simulink model "IEEE9BusSystem_1_1"  (R2025a)
settings: Solver=FixedStepDiscrete  StartTime=0.0  StopTime=20  FixedStep=Ts  RelTol=1e-3  AbsTol=1e-3  EnableMultiTasking=on
PreLoadFcn:
  | Ts = 1/60;
libraries: ee_lib x50, nesl_utility x29, fl_lib x22, eeGeneralControl x6, eeSmAC1C x3, eeSmPSS1A x3
(part 1 of 2)
Description:
  | IEEE 9-Bus System
settings Model: Creator=The MathWorks, Inc.  LastModifiedBy=Vishal
settings SolverCC: AutoScaleAbsTol=off  AlgebraicLoopSolver=TrustRegion
settings DataIOCC: MaxDataPoints=110000  SaveOutput=off  DSMLogging=off  SaveTime=off  ReturnWorkspaceOutputs=off  SignalLoggingName=logsout_IEEE9BusLoadflow
settings OptimizationCC: ReuseModelBlockBuffer=off  LifeSpan=inf
settings DebuggingCC: UnderspecifiedInitializationDetection=Classic  MergeDetectMultiDrivingBlocksExec=none  MaxConsecutiveZCsMsg=warning  UnconnectedInputMsg=warning  UnconnectedOutputMsg=warning  UnconnectedLineMsg=warning  SFUnexpectedBacktrackingDiag=warning  SFNoUnconditionalDefaultTransitionDiag=warning  SFExecutionAtInitializationDiag=none  ArithmeticOperatorsInVariantConditions=warning
settings ModelReferenceCC: EnableRefExpFcnMdlSchedulingChecks=on
settings SFSimCC: SimUseLocalCustomCode=off
settings RTWCC: RTWUseLocalCustomCode=off  GPUComputeCapability=3.5
settings CodeAppCC: StateflowObjectComments=on
settings GRTTargetCC: TargetLangStandard=C89/C90 (ANSI)
settings ConfigComp: CovMetricSettings=dw  CovSaveCumulativeToWorkspaceVar=on  CovSaveSingleToWorkspaceVar=on  CovExternalEMLEnable=off
settings SimscapeCC: SimscapeNormalizeSystem=off  SimscapeLogType=all  SimscapeLogName=simlog_IEEE9BusSystem  SimscapeLogLimitData=off  SimscapeOperatingPoint=op

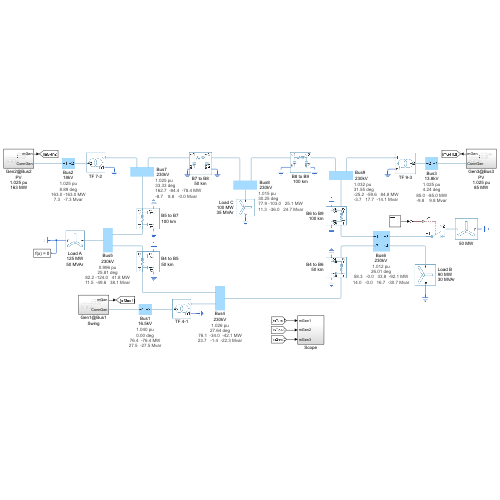
[thumbnail: Simulink's stored preview of the top-level diagram]
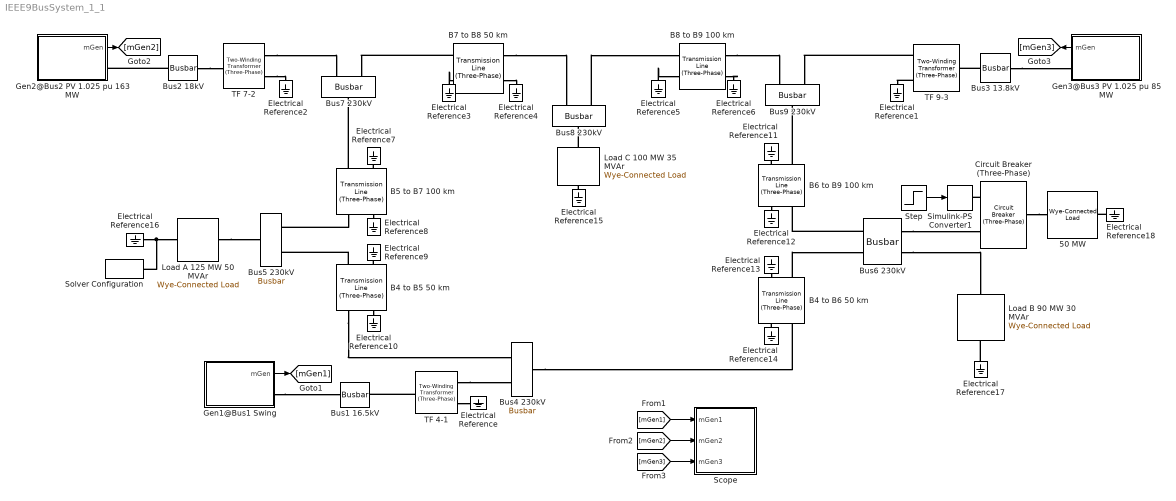
== system IEEE9BusSystem_1_1 ==
  50 MW : ee_lib/Passive/RLC Assemblies/Wye-Connected Load  port_option=ee.enum.threePhasePort.composite  parameterization=2  component_structure=1  component_structure_PQ=1  R=1 Ohm  L=0.001 H  C=1e-6 F  VRated=230 kV  FRated=60 Hz  P=50 MW  Qpos=30e6 V*A  Qneg=-100 V*A  R_parasitic=1e-6 Ohm  G_parasitic=1e-6 1/Ohm  R_parasitic_PQ=1e-6 Ohm  G_parasitic_PQ=1e-6*0 1/Ohm  Vmag0=230e3 V  Vang0=0 rad  Freq0=60 Hz  IL_specify=on  IL_priority=High  IL=[ 0 0 0 ] A  IL_nominal_specify=off  IL_nominal_value=1  IL_nominal_unit=A  VC_specify=on  VC_priority=High  VC=[ 0 0 0 ] V  VC_nominal_specify=off  VC_nominal_value=1  VC_nominal_unit=V
  B4 to B5 50 km : ee_lib/Passive/Lines/Transmission Line (Three-Phase)  length=50 km  freq=60 Hz  R=0.199333 Ohm/km  L=2.9658 mH/km  M=0.5803 mH/km  Cl=3.300e-3 uF/km  Cg=7.751e-3 uF/km  Rm=0.093533 Ohm/km  ModelTwoSections=ee.enum.enable.no  N=1  InterfacePosition=1 km  N1sec=1  N2sec=1  Access_ground=ee.enum.enable.no  R_parasitic=1e-6 Ohm  G_parasitic=1e-6 1/Ohm
      settings: InternalSimscapePortConfiguration="{\"Bottom\":[],\"Left\":[{\"id\":\"N1\",\"label\":\"~1\",\"type\":\"foundation.electrical.three_phase\"},{\"id\":\"g1\",\"label\":\"g1\",\"type\":\"foundation.electrical.electrical\"}],\"Right\":[{\"id\":\"N2\",\"label\":\"~2\",\"type\":\"foundation.electrical.three_phase\"},{\"id\":\"g2\",\"label\":\"g2\",\"type\":\"foundation.electrical.electrical\"}],\"Top\":[]}"
  B4 to B6 50 km : ee_lib/Passive/Lines/Transmission Line (Three-Phase)  length=50 km  freq=60 Hz  R=0.248707 Ohm/km  L=3.0967 mH/km  M=0.5148 mH/km  Cl=2.698e-3 uF/km  Cg=7.751e-3 uF/km  Rm=0.068847 Ohm/km  ModelTwoSections=ee.enum.enable.no  N=1  InterfacePosition=1 km  N1sec=1  N2sec=1  Access_ground=ee.enum.enable.no  R_parasitic=1e-6 Ohm  G_parasitic=1e-6 1/Ohm
      settings: InternalSimscapePortConfiguration="{\"Bottom\":[],\"Left\":[{\"id\":\"N1\",\"label\":\"~1\",\"type\":\"foundation.electrical.three_phase\"},{\"id\":\"g1\",\"label\":\"g1\",\"type\":\"foundation.electrical.electrical\"}],\"Right\":[{\"id\":\"N2\",\"label\":\"~2\",\"type\":\"foundation.electrical.three_phase\"},{\"id\":\"g2\",\"label\":\"g2\",\"type\":\"foundation.electrical.electrical\"}],\"Top\":[]}"
  B5 to B7 100 km : ee_lib/Passive/Lines/Transmission Line (Three-Phase)  length=100 km  freq=60 Hz  R=0.24165 Ohm/km  L=2.8816 mH/km  M=0.6224 mH/km  Cl=2.531e-3 uF/km  Cg=7.751e-3 uF/km  Rm=0.07237 Ohm/km  ModelTwoSections=ee.enum.enable.no  N=1  InterfacePosition=1 km  N1sec=1  N2sec=1  Access_ground=ee.enum.enable.no  R_parasitic=1e-6 Ohm  G_parasitic=1e-6 1/Ohm
      settings: InternalSimscapePortConfiguration="{\"Bottom\":[],\"Left\":[{\"id\":\"N1\",\"label\":\"~1\",\"type\":\"foundation.electrical.three_phase\"},{\"id\":\"g1\",\"label\":\"g1\",\"type\":\"foundation.electrical.electrical\"}],\"Right\":[{\"id\":\"N2\",\"label\":\"~2\",\"type\":\"foundation.electrical.three_phase\"},{\"id\":\"g2\",\"label\":\"g2\",\"type\":\"foundation.electrical.electrical\"}],\"Top\":[]}"
  B6 to B9 100 km : ee_lib/Passive/Lines/Transmission Line (Three-Phase)  length=100 km  freq=60 Hz  R=0.26634 Ohm/km  L=2.9658 mH/km  M=0.5803 mH/km  Cl=3.400e-3 uF/km  Cg=7.751e-3 uF/km  Rm=0.06003 Ohm/km  ModelTwoSections=ee.enum.enable.no  N=1  InterfacePosition=1 km  N1sec=1  N2sec=1  Access_ground=ee.enum.enable.no  R_parasitic=1e-6 Ohm  G_parasitic=1e-6 1/Ohm
      settings: InternalSimscapePortConfiguration="{\"Bottom\":[],\"Left\":[{\"id\":\"N1\",\"label\":\"~1\",\"type\":\"foundation.electrical.three_phase\"},{\"id\":\"g1\",\"label\":\"g1\",\"type\":\"foundation.electrical.electrical\"}],\"Right\":[{\"id\":\"N2\",\"label\":\"~2\",\"type\":\"foundation.electrical.three_phase\"},{\"id\":\"g2\",\"label\":\"g2\",\"type\":\"foundation.electrical.electrical\"}],\"Top\":[]}"
  B7 to B8 50 km : ee_lib/Passive/Lines/Transmission Line (Three-Phase)  length=50 km  freq=60 Hz  R=0.18875 Ohm/km  L=2.7226 mH/km  M=0.7019 mH/km  Cl=2.731e-3 uF/km  Cg=6.751e-3 uF/km  Rm=0.09882 Ohm/km  ModelTwoSections=ee.enum.enable.no  N=1  InterfacePosition=1 km  N1sec=1  N2sec=1  Access_ground=ee.enum.enable.no  R_parasitic=1e-6 Ohm  G_parasitic=1e-6 1/Ohm
      settings: InternalSimscapePortConfiguration="{\"Bottom\":[],\"Left\":[{\"id\":\"N1\",\"label\":\"~1\",\"type\":\"foundation.electrical.three_phase\"},{\"id\":\"g1\",\"label\":\"g1\",\"type\":\"foundation.electrical.electrical\"}],\"Right\":[{\"id\":\"N2\",\"label\":\"~2\",\"type\":\"foundation.electrical.three_phase\"},{\"id\":\"g2\",\"label\":\"g2\",\"type\":\"foundation.electrical.electrical\"}],\"Top\":[]}"
  B8 to B9 100 km : ee_lib/Passive/Lines/Transmission Line (Three-Phase)  length=100 km  freq=60 Hz  R=0.17077 Ohm/km  L=2.3184 mH/km  M=0.9040 mH/km  Cl=9.097e-4 uF/km  Cg=7.751e-3 uF/km  Rm=0.10782 Ohm/km  ModelTwoSections=ee.enum.enable.no  N=1  InterfacePosition=1 km  N1sec=1  N2sec=1  Access_ground=ee.enum.enable.no  R_parasitic=1e-6 Ohm  G_parasitic=1e-6 1/Ohm
      settings: InternalSimscapePortConfiguration="{\"Bottom\":[],\"Left\":[{\"id\":\"N1\",\"label\":\"~1\",\"type\":\"foundation.electrical.three_phase\"},{\"id\":\"g1\",\"label\":\"g1\",\"type\":\"foundation.electrical.electrical\"}],\"Right\":[{\"id\":\"N2\",\"label\":\"~2\",\"type\":\"foundation.electrical.three_phase\"},{\"id\":\"g2\",\"label\":\"g2\",\"type\":\"foundation.electrical.electrical\"}],\"Top\":[]}"
  Bus1 16.5kV : ee_lib/Connectors & References/Busbar  Tag="1.040 pu\\n0.00 deg\\n76.4  -76.4 MW\\n27.5  -27.5 Mvar"  n_nodes=ee.enum.connectors.busbar_number_of_connections.two  VRated=16.5 kV  freq=60 Hz  show_ps=ee.enum.connectors.busbar_measurement.false
      settings: AttributesFormatString=%<Tag>  InternalSimscapePortConfiguration="{\"Bottom\":[],\"Left\":[{\"id\":\"N1\",\"label\":\"~1\",\"type\":\"foundation.electrical.three_phase\"}],\"Right\":[{\"id\":\"N2\",\"label\":\"~2\",\"type\":\"foundation.electrical.three_phase\"}],\"Top\":[]}"
  Bus2 18kV : ee_lib/Connectors & References/Busbar  Tag="1.025 pu\\n8.89 deg\\n163.0 -163.0 MW\\n7.3   -7.3 Mvar"  n_nodes=ee.enum.connectors.busbar_number_of_connections.two  VRated=18 kV  freq=60 Hz  show_ps=ee.enum.connectors.busbar_measurement.false
      settings: AttributesFormatString=%<Tag>  InternalSimscapePortConfiguration="{\"Bottom\":[],\"Left\":[{\"id\":\"N1\",\"label\":\"~1\",\"type\":\"foundation.electrical.three_phase\"}],\"Right\":[{\"id\":\"N2\",\"label\":\"~2\",\"type\":\"foundation.electrical.three_phase\"}],\"Top\":[]}"
  Bus3 13.8kV : ee_lib/Connectors & References/Busbar  Tag="1.025 pu\\n4.24 deg\\n85.0  -85.0 MW\\n-9.8    9.8 Mvar"  n_nodes=ee.enum.connectors.busbar_number_of_connections.two  VRated=13.8 kV  freq=60 Hz  show_ps=ee.enum.connectors.busbar_measurement.false
      settings: AttributesFormatString=%<Tag>  InternalSimscapePortConfiguration="{\"Bottom\":[],\"Left\":[{\"id\":\"N1\",\"label\":\"~1\",\"type\":\"foundation.electrical.three_phase\"}],\"Right\":[{\"id\":\"N2\",\"label\":\"~2\",\"type\":\"foundation.electrical.three_phase\"}],\"Top\":[]}"
  Bus4 230kV : ee_lib/Connectors & References/Busbar  Tag="1.026 pu\\n27.64 deg\\n76.1  -34.0  -42.1 MW\\n23.7   -1.4  -22.3 Mvar"  n_nodes=ee.enum.connectors.busbar_number_of_connections.three  VRated=230 kV  freq=60 Hz  show_ps=ee.enum.connectors.busbar_measurement.false
      settings: AttributesFormatString=%<Tag>  InternalSimscapePortConfiguration="{\"Bottom\":[],\"Left\":[{\"id\":\"N1\",\"label\":\"~1\",\"type\":\"foundation.electrical.three_phase\"},{\"id\":\"N3\",\"label\":\"~3\",\"type\":\"foundation.electrical.three_phase\"}],\"Right\":[{\"id\":\"N2\",\"label\":\"~2\",\"type\":\"foundation.electrical.three_phase\"}],\"Top\":[]}"
  Bus5 230kV : ee_lib/Connectors & References/Busbar  Tag="0.996 pu\\n25.81 deg\\n82.2 -124.0   41.8 MW\\n11.5  -49.6   38.1 Mvar"  n_nodes=ee.enum.connectors.busbar_number_of_connections.three  VRated=230 kV  freq=60 Hz  show_ps=ee.enum.connectors.busbar_measurement.false
      settings: AttributesFormatString=%<Tag>  InternalSimscapePortConfiguration="{\"Bottom\":[],\"Left\":[{\"id\":\"N1\",\"label\":\"~1\",\"type\":\"foundation.electrical.three_phase\"},{\"id\":\"N3\",\"label\":\"~3\",\"type\":\"foundation.electrical.three_phase\"}],\"Right\":[{\"id\":\"N2\",\"label\":\"~2\",\"type\":\"foundation.electrical.three_phase\"}],\"Top\":[]}"
  Bus6 230kV : ee_lib/Connectors & References/Busbar  Tag="1.012 pu\\n26.01 deg\\n58.3   -0.0   33.8  -92.1 MW\\n14.0   -0.0   16.7  -30.7 Mvar"  n_nodes=ee.enum.connectors.busbar_number_of_connections.four  VRated=230 kV  freq=60 Hz  show_ps=ee.enum.connectors.busbar_measurement.false
      settings: AttributesFormatString=%<Tag>  InternalSimscapePortConfiguration="{\"Bottom\":[],\"Left\":[{\"id\":\"N1\",\"label\":\"~1\",\"type\":\"foundation.electrical.three_phase\"},{\"id\":\"N3\",\"label\":\"~3\",\"type\":\"foundation.electrical.three_phase\"}],\"Right\":[{\"id\":\"N2\",\"label\":\"~2\",\"type\":\"foundation.electrical.three_phase\"},{\"id\":\"N4\",\"label\":\"~4\",\"type\":\"foundation.electrical.three_phase\"}],\"Top\":[]}"
  Bus7 230kV : ee_lib/Connectors & References/Busbar  Tag="1.025 pu\\n33.33 deg\\n162.7  -84.4  -78.4 MW\\n-8.7    8.8   -0.0 Mvar"  n_nodes=ee.enum.connectors.busbar_number_of_connections.three  VRated=230 kV  freq=60 Hz  show_ps=ee.enum.connectors.busbar_measurement.false
      settings: AttributesFormatString=%<Tag>  InternalSimscapePortConfiguration="{\"Bottom\":[],\"Left\":[{\"id\":\"N1\",\"label\":\"~1\",\"type\":\"foundation.electrical.three_phase\"},{\"id\":\"N3\",\"label\":\"~3\",\"type\":\"foundation.electrical.three_phase\"}],\"Right\":[{\"id\":\"N2\",\"label\":\"~2\",\"type\":\"foundation.electrical.three_phase\"}],\"Top\":[]}"
  Bus8 230kV : ee_lib/Connectors & References/Busbar  Tag="1.015 pu\\n30.25 deg\\n77.9 -103.0   25.1 MW\\n11.3  -36.0   24.7 Mvar"  n_nodes=ee.enum.connectors.busbar_number_of_connections.three  VRated=230 kV  freq=60 Hz  show_ps=ee.enum.connectors.busbar_measurement.false
      settings: AttributesFormatString=%<Tag>  InternalSimscapePortConfiguration="{\"Bottom\":[],\"Left\":[{\"id\":\"N1\",\"label\":\"~1\",\"type\":\"foundation.electrical.three_phase\"},{\"id\":\"N3\",\"label\":\"~3\",\"type\":\"foundation.electrical.three_phase\"}],\"Right\":[{\"id\":\"N2\",\"label\":\"~2\",\"type\":\"foundation.electrical.three_phase\"}],\"Top\":[]}"
  Bus9 230kV : ee_lib/Connectors & References/Busbar  Tag="1.032 pu\\n31.55 deg\\n-25.2  -59.6   84.8 MW\\n-3.7   17.7  -14.1 Mvar"  n_nodes=ee.enum.connectors.busbar_number_of_connections.three  VRated=230 kV  freq=60 Hz  show_ps=ee.enum.connectors.busbar_measurement.false
      settings: AttributesFormatString=%<Tag>  InternalSimscapePortConfiguration="{\"Bottom\":[],\"Left\":[{\"id\":\"N1\",\"label\":\"~1\",\"type\":\"foundation.electrical.three_phase\"},{\"id\":\"N3\",\"label\":\"~3\",\"type\":\"foundation.electrical.three_phase\"}],\"Right\":[{\"id\":\"N2\",\"label\":\"~2\",\"type\":\"foundation.electrical.three_phase\"}],\"Top\":[]}"
  Circuit Breaker (Three-Phase) : ee_lib/Switches & Breakers/Circuit Breaker (Three-Phase)  R_closed=0.001 Ohm  G_open=1e-8 1/Ohm  threshold=0.5 V  breaker_behavior=ee.enum.switches.breakerBehavior.zeroCrossingDisable
      settings: InternalSimscapePortConfiguration="{\"Bottom\":[],\"Left\":[{\"id\":\"vT\",\"label\":\"vT\",\"type\":\"input\"},{\"id\":\"N1\",\"label\":\"~1\",\"type\":\"foundation.electrical.three_phase\"}],\"Right\":[{\"id\":\"N2\",\"label\":\"~2\",\"type\":\"foundation.electrical.three_phase\"}],\"Top\":[]}"
  Electrical Reference{,1..18} (19 alike) : fl_lib/Electrical/Electrical Elements/Electrical Reference
  Gen1@Bus1 Swing : Subsystem
  Gen2@Bus2 PV 1.025 pu 163 MW : Subsystem
  Gen3@Bus3 PV 1.025 pu 85 MW : Subsystem
  Load A 125 MW 50 MVAr : ee_lib/Passive/RLC Assemblies/Wye-Connected Load  port_option=ee.enum.threePhasePort.composite  parameterization=2  component_structure=1  component_structure_PQ=4  R=1 Ohm  L=0.001 H  C=1e-6 F  VRated=230e3 V  FRated=60 Hz  P=125e6 W  Qpos=50e6 V*A  Qneg=-100 V*A  R_parasitic=1e-6 Ohm  G_parasitic=1e-6 1/Ohm  R_parasitic_PQ=1e-6 Ohm  G_parasitic_PQ=1e-6 1/Ohm  Vmag0=230e3 V  Vang0=0 deg  Freq0=60 Hz  IL_specify=on  IL_priority=High  IL=[ 0 0 0 ] A  IL_nominal_specify=off  IL_nominal_value=1  IL_nominal_unit=A  VC_specify=on  VC_priority=High  VC=[ 0 0 0 ] V  VC_nominal_specify=off  VC_nominal_value=1  VC_nominal_unit=V
  Load B 90 MW 30 MVAr : ee_lib/Passive/RLC Assemblies/Wye-Connected Load  port_option=ee.enum.threePhasePort.composite  parameterization=2  component_structure=1  component_structure_PQ=4  R=1 Ohm  L=0.001 H  C=1e-6 F  VRated=230e3 V  FRated=60 Hz  P=90e6 W  Qpos=30e6 V*A  Qneg=-100 V*A  R_parasitic=1e-6 Ohm  G_parasitic=1e-6 1/Ohm  R_parasitic_PQ=1e-6 Ohm  G_parasitic_PQ=1e-6*0 1/Ohm  Vmag0=230e3 V  Vang0=0 deg  Freq0=60 Hz  IL_specify=on  IL_priority=High  IL=[ 0 0 0 ] A  IL_nominal_specify=off  IL_nominal_value=1  IL_nominal_unit=A  VC_specify=on  VC_priority=High  VC=[ 0 0 0 ] V  VC_nominal_specify=off  VC_nominal_value=1  VC_nominal_unit=V
  Load C 100 MW 35 MVAr : ee_lib/Passive/RLC Assemblies/Wye-Connected Load  port_option=ee.enum.threePhasePort.composite  parameterization=2  component_structure=1  component_structure_PQ=4  R=1 Ohm  L=0.001 H  C=1e-6 F  VRated=230e3 V  FRated=60 Hz  P=100e6 W  Qpos=35e6 V*A  Qneg=-100 V*A  R_parasitic=1e-6 Ohm  G_parasitic=1e-6 1/Ohm  R_parasitic_PQ=1e-6 Ohm  G_parasitic_PQ=1e-6 1/Ohm  Vmag0=230e3 V  Vang0=0 deg  Freq0=60 Hz  IL_specify=on  IL_priority=High  IL=[ 0 0 0 ] A  IL_nominal_specify=off  IL_nominal_value=1  IL_nominal_unit=A  VC_specify=on  VC_priority=High  VC=[ 0 0 0 ] V  VC_nominal_specify=off  VC_nominal_value=1  VC_nominal_unit=V
  Scope : Subsystem
  Simulink-PS Converter1 : nesl_utility/Simulink-PS Converter  PhysicalDomain=network_engine_domain  SubClassName=ps_input  LeftPortType=input  RightPortType=output  PseudoPeriodic=off  Frequencies=[]  NoiseDistribution=none  NoiseParameters=[]  Unit=1  AffineConversion=off  FilteringAndDerivatives=provide  SimscapeFilterOrder=1  InputFilterTimeConstant=0.001  UdotUserProvided=0
  Solver Configuration : nesl_utility/Solver Configuration  PhysicalDomain=network_engine_domain  SubClassName=solver  LeftPortType=input  RightPortType=generic  Tones=[]  Harmonics=[]  SimulateNoise=off  Profile=off  UseLocalSampling=off  EnableSwitchedLinearOptims=on  FrequencyDomain=off  UseCCode=off  RelTol=0.001  AbsTol=1e-06  MinStep=1e-09  ToWorkspace=off  RevertToSquareIcSolve=off  NumHomotopyIterations=100  PhasorMode=off  PhasorModeNumHarmonics=1  ConsistencySolver=NEWTON_FTOL  IndexReductionMethod=DerivativeReplacement  DoDC=off  ResidualTolerance=1e-09  ConsistencyTolSource=GLOBAL  ConsistencyAbsTol=0.001  ConsistencyRelTol=0.001  ConsistencyTolFactor=0.001  UseLocalSolver=on  LocalSolverChoice=NE_BACKWARD_EULER_ADVANCER  ResolveIndetEquations=on  FunctionEvalNumThread=1  LocalSolverSampleTime=Ts  DoFixedCost=on  MaxNonlinIter=3  MaxModeIter=2  ComputeImpulses=off  ImpulseIterations=2  LinearAlgebra=auto  LinearAlgebraNumThread=0  EquationFormulation=NE_FREQUENCY_TIME_EF  DelaysMemoryBudget=1024  AutomaticFiltering=on  FilteringTimeConstant=0.001  PartitionStorageMethod=AS_NEEDED  PartitionMemoryBudget=1024  PartitionMethod=FAST  MultibodyUseLocalSolver=off  MultibodyLocalSolverChoice=ODE1  MultibodyLocalSolverSampleTime=0.001
  Step : Step  Time=10  Before=1  After=0  SampleTime=0
  TF 4-1 : ee_lib/Passive/Transformers/Two-Winding Transformer (Three-Phase)  SRated=100e6 V*A  FRated=60 Hz  Winding1Connection=ee.enum.windingconnection.Yn  VRated1=230e3 V  Winding2Connection=ee.enum.windingconnection.delta1  VRated2=16.5e3 V  CoreType=ee.enum.coretype.fivelimb  pu_Rw1=1e-4  pu_Rw2=1e-4  leakage_reactance_option=ee.enum.transformer_leakage.include  pu_Xl1=0.0576/2  pu_Xl2=0.0576/2  magnetizing_resistance_option=ee.enum.transformer_magnetizingResistance.include  pu_Rm=500  magnetizing_reactance_option=ee.enum.transformer_magnetizingReactance.include  saturation_option=ee.enum.transformer_saturation.exclude  pu_Xm=500  current_data=[0, .002, 1, 2]  magnetic_flux_data=[0, 1.2, 1.5, 1.51]  pu_X0=0.5  i1_specify=off  i1_priority=None  i1=[ 0 0 0 ] A  i1_nominal_specify=off  i1_nominal_value=1  i1_nominal_unit=A  i2_specify=off  i2_priority=None  i2=[ 0 0 0 ] A  i2_nominal_specify=off  i2_nominal_value=1  i2_nominal_unit=A  phi_specify=off  phi_priority=None  phi=[ 0 0 0 ]  phi_nominal_specify=off  phi_nominal_value=1  phi_nominal_unit=1  power_dissipated_specify=off  power_dissipated_priority=None  power_dissipated=0 W  power_dissipated_nominal_specify=off  power_dissipated_nominal_value=1  power_dissipated_nominal_unit=W
      settings: InternalSimscapePortConfiguration="{\"Bottom\":[],\"Left\":[{\"id\":\"N1\",\"label\":\"~1\",\"type\":\"foundation.electrical.three_phase\"},{\"id\":\"n1\",\"label\":\"n1\",\"type\":\"foundation.electrical.electrical\"}],\"Right\":[{\"id\":\"N2\",\"label\":\"~2\",\"type\":\"foundation.electrical.three_phase\"}],\"Top\":[]}"
  TF 7-2 : ee_lib/Passive/Transformers/Two-Winding Transformer (Three-Phase)  SRated=100e6 V*A  FRated=60 Hz  Winding1Connection=ee.enum.windingconnection.Yn  VRated1=230e3 V  Winding2Connection=ee.enum.windingconnection.delta1  VRated2=18e3 V  CoreType=ee.enum.coretype.fivelimb  pu_Rw1=1e-4  pu_Rw2=1e-4  leakage_reactance_option=ee.enum.transformer_leakage.include  pu_Xl1=0.0625/2  pu_Xl2=0.0625/2  magnetizing_resistance_option=ee.enum.transformer_magnetizingResistance.include  pu_Rm=500  magnetizing_reactance_option=ee.enum.transformer_magnetizingReactance.include  saturation_option=ee.enum.transformer_saturation.exclude  pu_Xm=500  current_data=[0, .002, 1, 2]  magnetic_flux_data=[0, 1.2, 1.5, 1.51]  pu_X0=0.5  i1_specify=off  i1_priority=None  i1=[ 0 0 0 ] A  i1_nominal_specify=off  i1_nominal_value=1  i1_nominal_unit=A  i2_specify=off  i2_priority=None  i2=[ 0 0 0 ] A  i2_nominal_specify=off  i2_nominal_value=1  i2_nominal_unit=A  phi_specify=off  phi_priority=None  phi=[ 0 0 0 ]  phi_nominal_specify=off  phi_nominal_value=1  phi_nominal_unit=1  power_dissipated_specify=off  power_dissipated_priority=None  power_dissipated=0 W  power_dissipated_nominal_specify=off  power_dissipated_nominal_value=1  power_dissipated_nominal_unit=W
      settings: InternalSimscapePortConfiguration="{\"Bottom\":[],\"Left\":[{\"id\":\"N1\",\"label\":\"~1\",\"type\":\"foundation.electrical.three_phase\"},{\"id\":\"n1\",\"label\":\"n1\",\"type\":\"foundation.electrical.electrical\"}],\"Right\":[{\"id\":\"N2\",\"label\":\"~2\",\"type\":\"foundation.electrical.three_phase\"}],\"Top\":[]}"
  TF 9-3 : ee_lib/Passive/Transformers/Two-Winding Transformer (Three-Phase)  SRated=100e6 V*A  FRated=60 Hz  Winding1Connection=ee.enum.windingconnection.Yn  VRated1=230e3 V  Winding2Connection=ee.enum.windingconnection.delta1  VRated2=13.8e3 V  CoreType=ee.enum.coretype.fivelimb  pu_Rw1=1e-4  pu_Rw2=1e-4  leakage_reactance_option=ee.enum.transformer_leakage.include  pu_Xl1=0.0586/2  pu_Xl2=0.0586/2  magnetizing_resistance_option=ee.enum.transformer_magnetizingResistance.include  pu_Rm=500  magnetizing_reactance_option=ee.enum.transformer_magnetizingReactance.include  saturation_option=ee.enum.transformer_saturation.exclude  pu_Xm=500  current_data=[0, .002, 1, 2]  magnetic_flux_data=[0, 1.2, 1.5, 1.51]  pu_X0=0.5  i1_specify=off  i1_priority=None  i1=[ 0 0 0 ] A  i1_nominal_specify=off  i1_nominal_value=1  i1_nominal_unit=A  i2_specify=off  i2_priority=None  i2=[ 0 0 0 ] A  i2_nominal_specify=off  i2_nominal_value=1  i2_nominal_unit=A  phi_specify=off  phi_priority=None  phi=[ 0 0 0 ]  phi_nominal_specify=off  phi_nominal_value=1  phi_nominal_unit=1  power_dissipated_specify=off  power_dissipated_priority=None  power_dissipated=0 W  power_dissipated_nominal_specify=off  power_dissipated_nominal_value=1  power_dissipated_nominal_unit=W
      settings: InternalSimscapePortConfiguration="{\"Bottom\":[],\"Left\":[{\"id\":\"N1\",\"label\":\"~1\",\"type\":\"foundation.electrical.three_phase\"},{\"id\":\"n1\",\"label\":\"n1\",\"type\":\"foundation.electrical.electrical\"}],\"Right\":[{\"id\":\"N2\",\"label\":\"~2\",\"type\":\"foundation.electrical.three_phase\"}],\"Top\":[]}"
  wires:
  Gen2@Bus2 PV 1.025 pu 163 MW/1(mGen) -> [mGen2]
  Gen1@Bus1 Swing/1(mGen) -> [mGen1]
  Gen3@Bus3 PV 1.025 pu 85 MW/1(mGen) -> [mGen3]
  Step/1 -> Simulink-PS Converter1/1
  [mGen1] -> Scope/1(mGen1)
  [mGen2] -> Scope/2(mGen2)
  [mGen3] -> Scope/3(mGen3)
  connections:
  Electrical Reference16/LConn1 -- Solver Configuration/RConn1 -- Load A 125 MW 50 MVAr/RConn1
  B6 to B9 100 km/RConn1 -- Bus9 230kV/RConn1
  B8 to B9 100 km/RConn1 -- Bus9 230kV/LConn1
  B7 to B8 50 km/RConn1 -- Bus8 230kV/LConn1
  B4 to B5 50 km/RConn1 -- Bus5 230kV/LConn2
  B5 to B7 100 km/LConn1 -- Bus5 230kV/LConn1
  Load A 125 MW 50 MVAr/LConn1 -- Bus5 230kV/RConn1
  B5 to B7 100 km/RConn1 -- Bus7 230kV/RConn1
  TF 7-2/LConn1 -- Bus7 230kV/LConn1
  B6 to B9 100 km/LConn2 -- Electrical Reference12/LConn1
  TF 4-1/LConn1 -- Bus4 230kV/LConn1
  Load C 100 MW 35 MVAr/LConn1 -- Bus8 230kV/RConn1
  Electrical Reference5/LConn1 -- B8 to B9 100 km/LConn2
  B7 to B8 50 km/RConn2 -- Electrical Reference4/LConn1
  Bus8 230kV/LConn2 -- B8 to B9 100 km/LConn1
  TF 7-2/LConn2 -- Electrical Reference2/LConn1
  TF 9-3/LConn1 -- Bus9 230kV/LConn2
  TF 4-1/LConn2 -- Electrical Reference/LConn1
  B5 to B7 100 km/RConn2 -- Electrical Reference7/LConn1
  B5 to B7 100 km/LConn2 -- Electrical Reference8/LConn1
  B8 to B9 100 km/RConn2 -- Electrical Reference6/LConn1
  TF 9-3/LConn2 -- Electrical Reference1/LConn1
  B4 to B5 50 km/RConn2 -- Electrical Reference9/LConn1
  Electrical Reference3/LConn1 -- B7 to B8 50 km/LConn2
  B4 to B5 50 km/LConn2 -- Electrical Reference10/LConn1
  Electrical Reference17/LConn1 -- Load B 90 MW 30 MVAr/RConn1
  B7 to B8 50 km/LConn1 -- Bus7 230kV/LConn2
  Electrical Reference15/LConn1 -- Load C 100 MW 35 MVAr/RConn1
  Bus4 230kV/RConn1 -- B4 to B6 50 km/LConn1
  B4 to B5 50 km/LConn1 -- Bus4 230kV/LConn2
  TF 4-1/RConn1 -- Bus1 16.5kV/RConn1
  Electrical Reference14/LConn1 -- B4 to B6 50 km/LConn2
  Electrical Reference13/LConn1 -- B4 to B6 50 km/RConn2
  Bus2 18kV/RConn1 -- TF 7-2/RConn1
  Bus6 230kV/LConn1 -- B6 to B9 100 km/LConn1
  B6 to B9 100 km/RConn2 -- Electrical Reference11/LConn1
  Bus2 18kV/LConn1 -- Gen2@Bus2 PV 1.025 pu 163 MW/RConn1
  Gen1@Bus1 Swing/RConn1 -- Bus1 16.5kV/LConn1
  Bus6 230kV/RConn2 -- Load B 90 MW 30 MVAr/LConn1
  Circuit Breaker (Three-Phase)/LConn1 -- Simulink-PS Converter1/RConn1
  Electrical Reference18/LConn1 -- 50 MW/RConn1
  Circuit Breaker (Three-Phase)/RConn1 -- 50 MW/LConn1
  Bus6 230kV/RConn1 -- Circuit Breaker (Three-Phase)/LConn2
  B4 to B6 50 km/RConn1 -- Bus6 230kV/LConn2
  Bus3 13.8kV/LConn1 -- Gen3@Bus3 PV 1.025 pu 85 MW/RConn1
  Bus3 13.8kV/RConn1 -- TF 9-3/RConn1

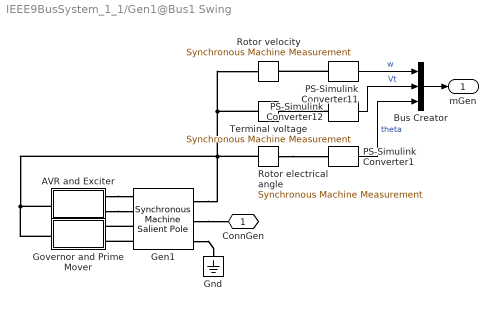
== system IEEE9BusSystem_1_1/Gen1@Bus1 Swing ==
  AVR and Exciter : Subsystem
  Bus Creator : BusCreator  Inputs=3
  Gen1 : ee_lib/Electromechanical/Synchronous/Synchronous Machine Salient Pole  port_option=ee.enum.threePhasePort.composite  SRated=247.5 MW  VRated=16.5 kV  FRated=60 Hz  nPolePairs=20  param_option=ee.enum.sm.parameterization.standard  fieldCircuitParameterization_option=ee.enum.sm.fieldparameterization.current  baseEfd=100 V  baseIfd=100 A  zero_sequence=ee.enum.park.zerosequence.include  axes_param=ee.enum.rotorangle.qaxis  Ladu=0.2725  Laqu=0.1510  L0=0.0888  Ll=0.0888  Ra=0.01  Lfd=0.0817  Rfd=1.0656e-4  L1d=0.0121  R1d=0.0039  L1q=0.0265  R1q=0.0052  Xl=0.0832  Xd=0.3614  Xq=0.2398  X0=0.0832  Xdd=0.1505  Xddd=0.0990  Xqdd=0.1114  d_option=ee.enum.circuit.open  Td0d=8.96 s  Tdd=1.75 s  Td0dd=0.05 s  Tddd=0.0214 s  q_option=ee.enum.circuit.open  Tq0dd=0.09 s  Tqdd=0.0232 s  saturation_option=ee.enum.saturation.exclude  saturation_ifd=[0.0, 0.48, 0.76, 1.38, 1.79]  saturation_Vag=[0.0, 0.43, 0.59, 0.71, 0.76]  initialization_option=ee.enum.sm.initialization.steadystate  source_type=ee.enum.sm.load_flow_source_type.Swing  Vmag0=16.5*1.04 kV  Vang0=0 deg  Pt0=100e6 V*A  Qt0=0 V*A  minimum_pu=0.95  phase_search_range=[-30, 30] deg  gmin=1e-6 S  connection_option=ee.enum.Connection.wye  num_q_dampers=1  rotor_offset=-pi / 2 rad  pu_psid_specify=on  pu_psid_priority=High  pu_psid=0  pu_psid_nominal_specify=off  pu_psid_nominal_value=1  pu_psid_nominal_unit=1  pu_psiq_specify=on  pu_psiq_priority=High  pu_psiq=0  pu_psiq_nominal_specify=off  pu_psiq_nominal_value=1  pu_psiq_nominal_unit=1  pu_psifd_specify=on  pu_psifd_priority=High  pu_psifd=0  pu_psifd_nominal_specify=off  pu_psifd_nominal_value=1  pu_psifd_nominal_unit=1  pu_psi1d_specify=on  pu_psi1d_priority=High  pu_psi1d=0  pu_psi1d_nominal_specify=off  pu_psi1d_nominal_value=1  pu_psi1d_nominal_unit=1  pu_psi1q_specify=on  pu_psi1q_priority=High  pu_psi1q=0  pu_psi1q_nominal_specify=off  pu_psi1q_nominal_value=1  pu_psi1q_nominal_unit=1  angular_position_diff_specify=on  angular_position_diff_priority=High  angular_position_diff=-86.2419 deg  angular_position_diff_nominal_specify=off  angular_position_diff_nominal_value=1  angular_position_diff_nominal_unit=deg  Tmeas=298.15 K  alpha=3.93e-3 1/K  stator_thermal_mass=100 J/K  rotor_thermal_mass=200 J/K  temperatureA_specify=off  temperatureA_priority=High  temperatureA=25 degC  temperatureA_nominal_specify=off  temperatureA_nominal_value=1  temperatureA_nominal_unit=degC  temperatureB_specify=off  temperatureB_priority=High  temperatureB=25 degC  temperatureB_nominal_specify=off  temperatureB_nominal_value=1  temperatureB_nominal_unit=degC  temperatureC_specify=off  temperatureC_priority=High  temperatureC=25 degC  temperatureC_nominal_specify=off  temperatureC_nominal_value=1  temperatureC_nominal_unit=degC  temperatureR_specify=off  temperatureR_priority=High  temperatureR=25 degC  temperatureR_nominal_specify=off  temperatureR_nominal_value=1  temperatureR_nominal_unit=degC
      settings: InternalSimscapePortConfiguration="{\"Bottom\":[],\"Left\":[{\"id\":\"fd_p\",\"label\":\"fd+\",\"type\":\"foundation.electrical.electrical\"},{\"id\":\"fd_n\",\"label\":\"fd-\",\"type\":\"foundation.electrical.electrical\"},{\"id\":\"R\",\"label\":\"R\",\"type\":\"foundation.mechanical.rotational.rotational\"},{\"id\":\"C\",\"label\":\"C\",\"type\":\"foundation.mechanical.rotational.rotational\"}],\"Right\":[{\"id\":\"pu_output\",\"label\":\"pu\",\"type\":\"output\"},{\"id\":\"N\",\"label\":\"~\",\"type\":\"foundation.electrical.three_phase\"},{\"id\":\"n\",\"label\":\"n\",\"type\":\"foundation.electrical.electrical\"}],\"Top\":[]}"
  Gnd : fl_lib/Electrical/Electrical Elements/Electrical Reference
  Governor and Prime Mover : Subsystem
  PS-Simulink Converter1 : nesl_utility/PS-Simulink Converter  PhysicalDomain=network_engine_domain  SubClassName=ps_output  LeftPortType=input  RightPortType=output  PseudoPeriodic=off  Frequencies=[]  VectorFormat=1-D array  Unit=1  AffineConversion=off
  PS-Simulink Converter11 : nesl_utility/PS-Simulink Converter  PhysicalDomain=network_engine_domain  SubClassName=ps_output  LeftPortType=input  RightPortType=output  PseudoPeriodic=off  Frequencies=[]  VectorFormat=1-D array  Unit=1  AffineConversion=off
  PS-Simulink Converter12 : nesl_utility/PS-Simulink Converter  PhysicalDomain=network_engine_domain  SubClassName=ps_output  LeftPortType=input  RightPortType=output  PseudoPeriodic=off  Frequencies=[]  VectorFormat=1-D array  Unit=1  AffineConversion=off
  Rotor electrical angle : ee_lib/Electromechanical/Synchronous/Synchronous Machine Measurement  output_idx=19
      settings: InternalSimscapePortConfiguration="{\"Bottom\":[],\"Left\":[{\"id\":\"pu_input\",\"label\":\"pu\",\"type\":\"input\"}],\"Right\":[{\"id\":\"pu_output\",\"label\":\"o\",\"type\":\"output\"}],\"Top\":[]}"
  Rotor velocity : ee_lib/Electromechanical/Synchronous/Synchronous Machine Measurement  output_idx=4
      settings: InternalSimscapePortConfiguration="{\"Bottom\":[],\"Left\":[{\"id\":\"pu_input\",\"label\":\"pu\",\"type\":\"input\"}],\"Right\":[{\"id\":\"pu_output\",\"label\":\"o\",\"type\":\"output\"}],\"Top\":[]}"
  Terminal voltage : ee_lib/Electromechanical/Synchronous/Synchronous Machine Measurement  output_idx=14
      settings: InternalSimscapePortConfiguration="{\"Bottom\":[],\"Left\":[{\"id\":\"pu_input\",\"label\":\"pu\",\"type\":\"input\"}],\"Right\":[{\"id\":\"pu_output\",\"label\":\"o\",\"type\":\"output\"}],\"Top\":[]}"
  ConnGen : PMIOPort  Side=Right
  mGen : Outport
  wires:
  PS-Simulink Converter1/1 -> Bus Creator/3  "theta"
  PS-Simulink Converter12/1 -> Bus Creator/2  "Vt"
  Bus Creator/1 -> mGen/1
  PS-Simulink Converter11/1 -> Bus Creator/1  "w"
  connections:
  Rotor electrical angle/RConn1 -- PS-Simulink Converter1/LConn1
  PS-Simulink Converter12/LConn1 -- Terminal voltage/RConn1
  PS-Simulink Converter11/LConn1 -- Rotor velocity/RConn1
  Rotor electrical angle/LConn1 -- Rotor velocity/LConn1 -- Terminal voltage/LConn1 -- Gen1/RConn1 -- AVR and Exciter/LConn1 -- Governor and Prime Mover/LConn1
  Gen1/RConn3 -- Gnd/LConn1
  Gen1/RConn2 -- ConnGen/RConn1
  Gen1/LConn4 -- Governor and Prime Mover/RConn2
  Gen1/LConn3 -- Governor and Prime Mover/RConn1
  AVR and Exciter/RConn2 -- Gen1/LConn2
  AVR and Exciter/RConn1 -- Gen1/LConn1

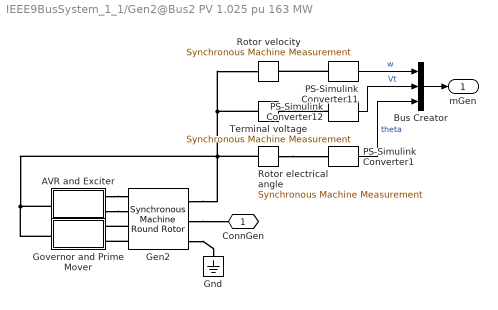
== system IEEE9BusSystem_1_1/Gen2@Bus2 PV 1.025 pu 163 MW ==
  AVR and Exciter : Subsystem
  Bus Creator : BusCreator  Inputs=3
  Gen2 : ee_lib/Electromechanical/Synchronous/Synchronous Machine Round Rotor  port_option=ee.enum.threePhasePort.composite  SRated=192 MW  VRated=18 kV  FRated=60 Hz  nPolePairs=1  param_option=ee.enum.sm.parameterization.standard  fieldCircuitParameterization_option=ee.enum.sm.fieldparameterization.current  baseEfd=92.95 V  baseIfd=100 A  zero_sequence=ee.enum.park.zerosequence.include  axes_param=ee.enum.rotorangle.qaxis  Ladu=1.6801  Laqu=1.62  L0=0.0399  Ll=0.0399  Ra=0.01  Lfd=0.2162  Rfd=8.558e-4  L1d=0.4343  R1d=0.0325  L1q=0.2635  R1q=0.0326  L2q=0.4627  R2q=0.0131  Xl=0.1  Xd=1.7199  Xq=1.6598  X0=0.1  Xdd=0.23  Xqd=0.378  Xddd=0.1728  Xqdd=0.192  d_option=ee.enum.circuit.open  Td0d=6 s  Tdd=1.3260 s  Td0dd=0.05 s  Tddd=0.0230 s  q_option=ee.enum.circuit.open  Tq0d=0.535 s  Tqd=0.3693 s  Tq0dd=0.04 s  Tqdd=0.0269 s  saturation_option=ee.enum.saturation.exclude  saturation_ifd=[0.0, 0.48, 0.76, 1.38, 1.79]  saturation_Vag=[0.0, 0.8, 1.08, 1.31, 1.4]  initialization_option=ee.enum.sm.initialization.steadystate  source_type=ee.enum.sm.load_flow_source_type.PV  Vmag0=18*1.025 kV  Vang0=0 deg  Pt0=163 MW  Qt0=0 V*A  minimum_pu=0.95  phase_search_range=[-30, 30] deg  gmin=1e-6 S  connection_option=ee.enum.Connection.wye  num_q_dampers=2  rotor_offset=-pi / 2 rad  pu_psid_specify=on  pu_psid_priority=High  pu_psid=0  pu_psid_nominal_specify=off  pu_psid_nominal_value=1  pu_psid_nominal_unit=1  pu_psiq_specify=on  pu_psiq_priority=High  pu_psiq=0  pu_psiq_nominal_specify=off  pu_psiq_nominal_value=1  pu_psiq_nominal_unit=1  pu_psifd_specify=on  pu_psifd_priority=High  pu_psifd=0  pu_psifd_nominal_specify=off  pu_psifd_nominal_value=1  pu_psifd_nominal_unit=1  pu_psi1d_specify=on  pu_psi1d_priority=High  pu_psi1d=0  pu_psi1d_nominal_specify=off  pu_psi1d_nominal_value=1  pu_psi1d_nominal_unit=1  pu_psi1q_specify=on  pu_psi1q_priority=High  pu_psi1q=0  pu_psi1q_nominal_specify=off  pu_psi1q_nominal_value=1  pu_psi1q_nominal_unit=1  pu_psi2q_specify=on  pu_psi2q_priority=High  pu_psi2q=0  pu_psi2q_nominal_specify=off  pu_psi2q_nominal_value=1  pu_psi2q_nominal_unit=1  angular_position_diff_specify=off  angular_position_diff_priority=None  angular_position_diff=0 deg  angular_position_diff_nominal_specify=off  angular_position_diff_nominal_value=1  angular_position_diff_nominal_unit=deg  Tmeas=298.15 K  alpha=3.93e-3 1/K  stator_thermal_mass=100 J/K  rotor_thermal_mass=200 J/K  temperatureA_specify=off  temperatureA_priority=High  temperatureA=25 degC  temperatureA_nominal_specify=off  temperatureA_nominal_value=1  temperatureA_nominal_unit=degC  temperatureB_specify=off  temperatureB_priority=High  temperatureB=25 degC  temperatureB_nominal_specify=off  temperatureB_nominal_value=1  temperatureB_nominal_unit=degC  temperatureC_specify=off  temperatureC_priority=High  temperatureC=25 degC  temperatureC_nominal_specify=off  temperatureC_nominal_value=1  temperatureC_nominal_unit=degC  temperatureR_specify=off  temperatureR_priority=High  temperatureR=25 degC  temperatureR_nominal_specify=off  temperatureR_nominal_value=1  temperatureR_nominal_unit=degC
      settings: InternalSimscapePortConfiguration="{\"Bottom\":[],\"Left\":[{\"id\":\"fd_p\",\"label\":\"fd+\",\"type\":\"foundation.electrical.electrical\"},{\"id\":\"fd_n\",\"label\":\"fd-\",\"type\":\"foundation.electrical.electrical\"},{\"id\":\"R\",\"label\":\"R\",\"type\":\"foundation.mechanical.rotational.rotational\"},{\"id\":\"C\",\"label\":\"C\",\"type\":\"foundation.mechanical.rotational.rotational\"}],\"Right\":[{\"id\":\"pu_output\",\"label\":\"pu\",\"type\":\"output\"},{\"id\":\"N\",\"label\":\"~\",\"type\":\"foundation.electrical.three_phase\"},{\"id\":\"n\",\"label\":\"n\",\"type\":\"foundation.electrical.electrical\"}],\"Top\":[]}"
  Gnd : fl_lib/Electrical/Electrical Elements/Electrical Reference
  Governor and Prime Mover : Subsystem
  PS-Simulink Converter1 : nesl_utility/PS-Simulink Converter  PhysicalDomain=network_engine_domain  SubClassName=ps_output  LeftPortType=input  RightPortType=output  PseudoPeriodic=off  Frequencies=[]  VectorFormat=1-D array  Unit=1  AffineConversion=off
  PS-Simulink Converter11 : nesl_utility/PS-Simulink Converter  PhysicalDomain=network_engine_domain  SubClassName=ps_output  LeftPortType=input  RightPortType=output  PseudoPeriodic=off  Frequencies=[]  VectorFormat=1-D array  Unit=1  AffineConversion=off
  PS-Simulink Converter12 : nesl_utility/PS-Simulink Converter  PhysicalDomain=network_engine_domain  SubClassName=ps_output  LeftPortType=input  RightPortType=output  PseudoPeriodic=off  Frequencies=[]  VectorFormat=1-D array  Unit=1  AffineConversion=off
  Rotor electrical angle : ee_lib/Electromechanical/Synchronous/Synchronous Machine Measurement  output_idx=19
      settings: InternalSimscapePortConfiguration="{\"Bottom\":[],\"Left\":[{\"id\":\"pu_input\",\"label\":\"pu\",\"type\":\"input\"}],\"Right\":[{\"id\":\"pu_output\",\"label\":\"o\",\"type\":\"output\"}],\"Top\":[]}"
  Rotor velocity : ee_lib/Electromechanical/Synchronous/Synchronous Machine Measurement  output_idx=4
      settings: InternalSimscapePortConfiguration="{\"Bottom\":[],\"Left\":[{\"id\":\"pu_input\",\"label\":\"pu\",\"type\":\"input\"}],\"Right\":[{\"id\":\"pu_output\",\"label\":\"o\",\"type\":\"output\"}],\"Top\":[]}"
  Terminal voltage : ee_lib/Electromechanical/Synchronous/Synchronous Machine Measurement  output_idx=14
      settings: InternalSimscapePortConfiguration="{\"Bottom\":[],\"Left\":[{\"id\":\"pu_input\",\"label\":\"pu\",\"type\":\"input\"}],\"Right\":[{\"id\":\"pu_output\",\"label\":\"o\",\"type\":\"output\"}],\"Top\":[]}"
  ConnGen : PMIOPort  Side=Right
  mGen : Outport
  wires:
  PS-Simulink Converter11/1 -> Bus Creator/1  "w"
  Bus Creator/1 -> mGen/1
  PS-Simulink Converter12/1 -> Bus Creator/2  "Vt"
  PS-Simulink Converter1/1 -> Bus Creator/3  "theta"
  connections:
  AVR and Exciter/RConn1 -- Gen2/LConn1
  AVR and Exciter/RConn2 -- Gen2/LConn2
  Gen2/LConn3 -- Governor and Prime Mover/RConn1
  Gen2/LConn4 -- Governor and Prime Mover/RConn2
  Gen2/RConn2 -- ConnGen/RConn1
  Gen2/RConn3 -- Gnd/LConn1
  Gen2/RConn1 -- AVR and Exciter/LConn1 -- Governor and Prime Mover/LConn1 -- Rotor electrical angle/LConn1 -- Rotor velocity/LConn1 -- Terminal voltage/LConn1
  PS-Simulink Converter11/LConn1 -- Rotor velocity/RConn1
  PS-Simulink Converter12/LConn1 -- Terminal voltage/RConn1
  Rotor electrical angle/RConn1 -- PS-Simulink Converter1/LConn1

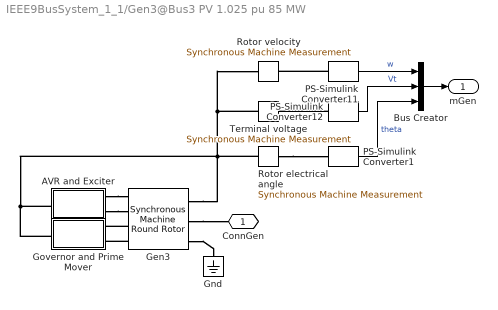
== system IEEE9BusSystem_1_1/Gen3@Bus3 PV 1.025 pu 85 MW ==
  AVR and Exciter : Subsystem
  Bus Creator : BusCreator  Inputs=3
  Gen3 : ee_lib/Electromechanical/Synchronous/Synchronous Machine Round Rotor  port_option=ee.enum.threePhasePort.composite  SRated=128 MW  VRated=13.8 kV  FRated=60 Hz  nPolePairs=1  param_option=ee.enum.sm.parameterization.standard  fieldCircuitParameterization_option=ee.enum.sm.fieldparameterization.current  baseEfd=92.95 V  baseIfd=100 A  zero_sequence=ee.enum.park.zerosequence.include  axes_param=ee.enum.rotorangle.qaxis  Ladu=1.5958  Laqu=1.5257  L0=0.0842  Ll=0.0842  Ra=0.01  Lfd=0.1715  Rfd=8.4749e-4  L1d=0.061  R1d=0.0108  L1q=0.1726  R1q=0.0222  L2q=0.3535  R2q=0.0144  Xl=0.095  Xd=1.68  Xq=1.61  X0=0.095  Xdd=0.2321  Xqd=0.32  Xddd=0.128  Xqdd=0.192  d_option=ee.enum.circuit.open  Td0d=5.89 s  Tdd=1.3260 s  Td0dd=0.05 s  Tddd=0.0230 s  q_option=ee.enum.circuit.open  Tq0d=0.6 s  Tqd=0.3693 s  Tq0dd=0.04 s  Tqdd=0.0269 s  saturation_option=ee.enum.saturation.exclude  saturation_ifd=[0.0, 0.48, 0.76, 1.38, 1.79]  saturation_Vag=[0.0, 0.8, 1.08, 1.31, 1.4]  initialization_option=ee.enum.sm.initialization.steadystate  source_type=ee.enum.sm.load_flow_source_type.PV  Vmag0=13.8*1.025 kV  Vang0=0 deg  Pt0=85 MW  Qt0=0 V*A  minimum_pu=0.95  phase_search_range=[-30, 30] deg  gmin=1e-6 S  connection_option=ee.enum.Connection.wye  num_q_dampers=2  rotor_offset=-pi / 2 rad  pu_psid_specify=on  pu_psid_priority=High  pu_psid=0  pu_psid_nominal_specify=off  pu_psid_nominal_value=1  pu_psid_nominal_unit=1  pu_psiq_specify=on  pu_psiq_priority=High  pu_psiq=0  pu_psiq_nominal_specify=off  pu_psiq_nominal_value=1  pu_psiq_nominal_unit=1  pu_psifd_specify=on  pu_psifd_priority=High  pu_psifd=0  pu_psifd_nominal_specify=off  pu_psifd_nominal_value=1  pu_psifd_nominal_unit=1  pu_psi1d_specify=on  pu_psi1d_priority=High  pu_psi1d=0  pu_psi1d_nominal_specify=off  pu_psi1d_nominal_value=1  pu_psi1d_nominal_unit=1  pu_psi1q_specify=on  pu_psi1q_priority=High  pu_psi1q=0  pu_psi1q_nominal_specify=off  pu_psi1q_nominal_value=1  pu_psi1q_nominal_unit=1  pu_psi2q_specify=on  pu_psi2q_priority=High  pu_psi2q=0  pu_psi2q_nominal_specify=off  pu_psi2q_nominal_value=1  pu_psi2q_nominal_unit=1  angular_position_diff_specify=off  angular_position_diff_priority=High  angular_position_diff=0 deg  angular_position_diff_nominal_specify=off  angular_position_diff_nominal_value=1  angular_position_diff_nominal_unit=deg  Tmeas=298.15 K  alpha=3.93e-3 1/K  stator_thermal_mass=100 J/K  rotor_thermal_mass=200 J/K  temperatureA_specify=off  temperatureA_priority=High  temperatureA=25 degC  temperatureA_nominal_specify=off  temperatureA_nominal_value=1  temperatureA_nominal_unit=degC  temperatureB_specify=off  temperatureB_priority=High  temperatureB=25 degC  temperatureB_nominal_specify=off  temperatureB_nominal_value=1  temperatureB_nominal_unit=degC  temperatureC_specify=off  temperatureC_priority=High  temperatureC=25 degC  temperatureC_nominal_specify=off  temperatureC_nominal_value=1  temperatureC_nominal_unit=degC  temperatureR_specify=off  temperatureR_priority=High  temperatureR=25 degC  temperatureR_nominal_specify=off  temperatureR_nominal_value=1  temperatureR_nominal_unit=degC
      settings: InternalSimscapePortConfiguration="{\"Bottom\":[],\"Left\":[{\"id\":\"fd_p\",\"label\":\"fd+\",\"type\":\"foundation.electrical.electrical\"},{\"id\":\"fd_n\",\"label\":\"fd-\",\"type\":\"foundation.electrical.electrical\"},{\"id\":\"R\",\"label\":\"R\",\"type\":\"foundation.mechanical.rotational.rotational\"},{\"id\":\"C\",\"label\":\"C\",\"type\":\"foundation.mechanical.rotational.rotational\"}],\"Right\":[{\"id\":\"pu_output\",\"label\":\"pu\",\"type\":\"output\"},{\"id\":\"N\",\"label\":\"~\",\"type\":\"foundation.electrical.three_phase\"},{\"id\":\"n\",\"label\":\"n\",\"type\":\"foundation.electrical.electrical\"}],\"Top\":[]}"
  Gnd : fl_lib/Electrical/Electrical Elements/Electrical Reference
  Governor and Prime Mover : Subsystem
  PS-Simulink Converter1 : nesl_utility/PS-Simulink Converter  PhysicalDomain=network_engine_domain  SubClassName=ps_output  LeftPortType=input  RightPortType=output  PseudoPeriodic=off  Frequencies=[]  VectorFormat=1-D array  Unit=1  AffineConversion=off
  PS-Simulink Converter11 : nesl_utility/PS-Simulink Converter  PhysicalDomain=network_engine_domain  SubClassName=ps_output  LeftPortType=input  RightPortType=output  PseudoPeriodic=off  Frequencies=[]  VectorFormat=1-D array  Unit=1  AffineConversion=off
  PS-Simulink Converter12 : nesl_utility/PS-Simulink Converter  PhysicalDomain=network_engine_domain  SubClassName=ps_output  LeftPortType=input  RightPortType=output  PseudoPeriodic=off  Frequencies=[]  VectorFormat=1-D array  Unit=1  AffineConversion=off
  Rotor electrical angle : ee_lib/Electromechanical/Synchronous/Synchronous Machine Measurement  output_idx=19
      settings: InternalSimscapePortConfiguration="{\"Bottom\":[],\"Left\":[{\"id\":\"pu_input\",\"label\":\"pu\",\"type\":\"input\"}],\"Right\":[{\"id\":\"pu_output\",\"label\":\"o\",\"type\":\"output\"}],\"Top\":[]}"
  Rotor velocity : ee_lib/Electromechanical/Synchronous/Synchronous Machine Measurement  output_idx=4
      settings: InternalSimscapePortConfiguration="{\"Bottom\":[],\"Left\":[{\"id\":\"pu_input\",\"label\":\"pu\",\"type\":\"input\"}],\"Right\":[{\"id\":\"pu_output\",\"label\":\"o\",\"type\":\"output\"}],\"Top\":[]}"
  Terminal voltage : ee_lib/Electromechanical/Synchronous/Synchronous Machine Measurement  output_idx=14
      settings: InternalSimscapePortConfiguration="{\"Bottom\":[],\"Left\":[{\"id\":\"pu_input\",\"label\":\"pu\",\"type\":\"input\"}],\"Right\":[{\"id\":\"pu_output\",\"label\":\"o\",\"type\":\"output\"}],\"Top\":[]}"
  ConnGen : PMIOPort  Side=Right
  mGen : Outport
  wires:
  PS-Simulink Converter1/1 -> Bus Creator/3  "theta"
  PS-Simulink Converter12/1 -> Bus Creator/2  "Vt"
  Bus Creator/1 -> mGen/1
  PS-Simulink Converter11/1 -> Bus Creator/1  "w"
  connections:
  Rotor electrical angle/RConn1 -- PS-Simulink Converter1/LConn1
  PS-Simulink Converter12/LConn1 -- Terminal voltage/RConn1
  PS-Simulink Converter11/LConn1 -- Rotor velocity/RConn1
  Terminal voltage/LConn1 -- Gen3/RConn1 -- Rotor electrical angle/LConn1 -- AVR and Exciter/LConn1 -- Governor and Prime Mover/LConn1 -- Rotor velocity/LConn1
  Gen3/RConn3 -- Gnd/LConn1
  Gen3/RConn2 -- ConnGen/RConn1
  Gen3/LConn4 -- Governor and Prime Mover/RConn2
  Gen3/LConn3 -- Governor and Prime Mover/RConn1
  AVR and Exciter/RConn2 -- Gen3/LConn2
  AVR and Exciter/RConn1 -- Gen3/LConn1

== system IEEE9BusSystem_1_1/Scope ==
  BusElementIn : Inport  PortName=mGen1  Element=w
  BusElementIn1 : Inport  PortName=mGen1  Element=Vt
  BusElementIn2 : Inport  Port=2  PortName=mGen2  Element=Vt
  BusElementIn4 : Inport  Port=2  PortName=mGen2  Element=w
  BusElementIn3 : Inport  Port=3  PortName=mGen3  Element=Vt
  BusElementIn5 : Inport  Port=3  PortName=mGen3  Element=w
  Mux : Mux  Inputs=3
  Mux1 : Mux  Inputs=3
  Scope : Scope  NumInputPorts=2
      settings: ActiveDisplayYMinimum=1.01012  ActiveDisplayYMaximum=1.04332
  wires:
  BusElementIn4/1 -> Mux/2
  BusElementIn/1 -> Mux/1
  BusElementIn5/1 -> Mux/3
  BusElementIn1/1 -> Mux1/1
  BusElementIn2/1 -> Mux1/2
  BusElementIn3/1 -> Mux1/3
  Mux1/1 -> Scope/1  "Terminal voltages [p.u.]"
  Mux/1 -> Scope/2  "Rotor speeds [p.u.]"

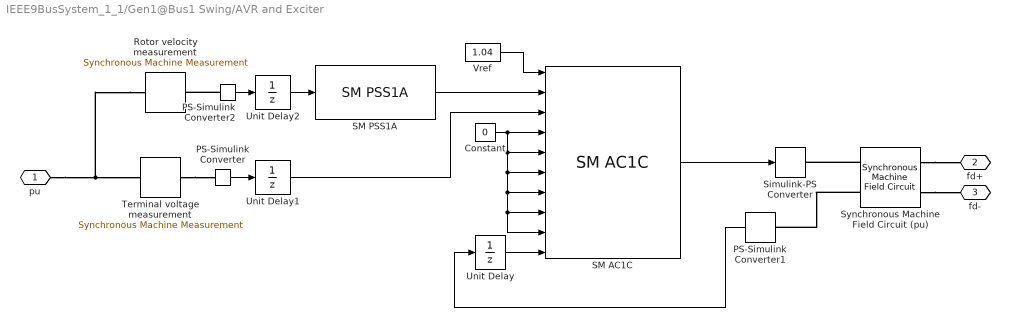
== system IEEE9BusSystem_1_1/Gen1@Bus1 Swing/AVR and Exciter ==
  Constant : Constant  Value=0
  PS-Simulink Converter : nesl_utility/PS-Simulink Converter  PhysicalDomain=network_engine_domain  SubClassName=ps_output  LeftPortType=input  RightPortType=output  PseudoPeriodic=off  Frequencies=[]  VectorFormat=1-D array  Unit=1  AffineConversion=off
  PS-Simulink Converter1 : nesl_utility/PS-Simulink Converter  PhysicalDomain=network_engine_domain  SubClassName=ps_output  LeftPortType=input  RightPortType=output  PseudoPeriodic=off  Frequencies=[]  VectorFormat=1-D array  Unit=1  AffineConversion=off
  PS-Simulink Converter2 : nesl_utility/PS-Simulink Converter  PhysicalDomain=network_engine_domain  SubClassName=ps_output  LeftPortType=input  RightPortType=output  PseudoPeriodic=off  Frequencies=[]  VectorFormat=1-D array  Unit=1  AffineConversion=off
  Rotor velocity measurement : ee_lib/Electromechanical/Synchronous/Synchronous Machine Measurement  output_idx=4
      settings: InternalSimscapePortConfiguration="{\"Bottom\":[],\"Left\":[{\"id\":\"pu_input\",\"label\":\"pu\",\"type\":\"input\"}],\"Right\":[{\"id\":\"pu_output\",\"label\":\"o\",\"type\":\"output\"}],\"Top\":[]}"
  SM AC1C : eeSmAC1C/SM AC1C  E_FD0=1.08614  Ts=Ts  R_C=0  X_C=0  T_R=0  K_A=400  T_A=0.02  T_B=0  T_C=0  K_F=0.03  T_F=1  V_Amax=14.5  V_Amin=-14.5  E_FEmax=6.03  E_FEmin=-5.43  oelInputLocation=Unused  uelInputLocation=Unused  sclInputLocation=Unused  K_E=1  T_E=0.8  K_C=0.2  K_D=0.38  E_1=4.18  S_E_E1=0.1  E_2=3.14  S_E_E2=0.03  V_FEmax=99  V_Emin=0
  SM PSS1A : eeSmPSS1A/SM PSS1A  K_S=3.15  A_1=0  A_2=0  T_1=0  T_2=0  T_3=0.32  T_4=0.016  T_5=1  T_6=0.0106  V_STmax=0.09  V_STmin=-0.09  Ts=Ts
  Simulink-PS Converter : nesl_utility/Simulink-PS Converter  PhysicalDomain=network_engine_domain  SubClassName=ps_input  LeftPortType=input  RightPortType=output  PseudoPeriodic=off  Frequencies=[]  NoiseDistribution=none  NoiseParameters=[]  Unit=1  AffineConversion=off  FilteringAndDerivatives=provide  SimscapeFilterOrder=1  InputFilterTimeConstant=0.001  UdotUserProvided=0
  Synchronous Machine Field Circuit (pu) : ee_lib/Electromechanical/Synchronous/Synchronous Machine Field Circuit  unit_option=ee.enum.unit.pu  SRated=247.5 MW  FRated=60 Hz  fieldCircuitParameterization_option=ee.enum.sm.fieldparameterization.current  baseEfd=92.95 V  baseIfd=100 A  parameterization_option=ee.enum.sm.parameterization.standard  Ladu=0.2725  Rfd=1.0656e-4  Xl=0.0832  Xd=0.3614  Xdd=0.1505  Xddd=0.0990  d_option=ee.enum.circuit.open  Td0d=8.96 s  Tdd=1.3260 s  Td0dd=0.05 s  Tddd=0.0230 s
      settings: InternalSimscapePortConfiguration="{\"Bottom\":[],\"Left\":[{\"id\":\"Efd_pu\",\"label\":\"Efd_pu\",\"type\":\"input\"},{\"id\":\"Ifd_pu\",\"label\":\"Ifd_pu\",\"type\":\"output\"}],\"Right\":[{\"id\":\"fd_p\",\"label\":\"fd+\",\"type\":\"foundation.electrical.electrical\"},{\"id\":\"fd_n\",\"label\":\"fd-\",\"type\":\"foundation.electrical.electrical\"}],\"Top\":[]}"
  Terminal voltage measurement : ee_lib/Electromechanical/Synchronous/Synchronous Machine Measurement  output_idx=14
      settings: InternalSimscapePortConfiguration="{\"Bottom\":[],\"Left\":[{\"id\":\"pu_input\",\"label\":\"pu\",\"type\":\"input\"}],\"Right\":[{\"id\":\"pu_output\",\"label\":\"o\",\"type\":\"output\"}],\"Top\":[]}"
  Unit Delay : UnitDelay  InitialCondition=1.08614  SampleTime=Ts  HasFrameUpgradeWarning=on
  Unit Delay1 : UnitDelay  InitialCondition=1.04  SampleTime=Ts  HasFrameUpgradeWarning=on
  Unit Delay2 : UnitDelay  InitialCondition=1  SampleTime=Ts  HasFrameUpgradeWarning=on
  Vref : Constant  Value=1.04
  pu : PMIOPort  Side=Left
  fd+ : PMIOPort  Port=2  Side=Right
  fd- : PMIOPort  Port=3  Side=Right
  wires:
  Unit Delay2/1 -> SM PSS1A/1
  PS-Simulink Converter2/1 -> Unit Delay2/1
  Unit Delay1/1 -> SM AC1C/3
  Vref/1 -> SM AC1C/1
  Constant/1 -> SM AC1C/9, SM AC1C/8, SM AC1C/7, SM AC1C/6, SM AC1C/5, SM AC1C/4
  Unit Delay/1 -> SM AC1C/10
  SM AC1C/1 -> Simulink-PS Converter/1
  PS-Simulink Converter1/1 -> Unit Delay/1
  SM PSS1A/1 -> SM AC1C/2
  PS-Simulink Converter/1 -> Unit Delay1/1
  connections:
  PS-Simulink Converter2/LConn1 -- Rotor velocity measurement/RConn1
  Rotor velocity measurement/LConn1 -- Terminal voltage measurement/LConn1 -- pu/RConn1
  Terminal voltage measurement/RConn1 -- PS-Simulink Converter/LConn1
  Synchronous Machine Field Circuit (pu)/LConn1 -- Simulink-PS Converter/RConn1
  Synchronous Machine Field Circuit (pu)/LConn2 -- PS-Simulink Converter1/LConn1
  Synchronous Machine Field Circuit (pu)/RConn2 -- fd-/RConn1
  Synchronous Machine Field Circuit (pu)/RConn1 -- fd+/RConn1
